simulink model "pitch_sim"  (R2025b)
settings: Solver=FixedStepAuto  StartTime=0.0  StopTime=15  FixedStep=0.0001  RelTol=1e-3
values from neighbouring files (symbols this model uses):
  A = [M1\M2; 0 0 1 0]    [Final_sim.m]    (also in hw2.m = 20; linear_fit_hw.m = [1 900 900^2; off_highway_tiremodel.m = [0.67 0.65 0.52 0.53 0.88]; sim3.m = [ 0 0 1 0)
  B = [M1\M3; 0 0]    [Final_sim.m]    (also in off_highway_tiremodel.m = 1.01*(100/Fz(1))*exp(0.14)-0.8401; sim3.m = [ 0     0; sim4.m = [(C1/m); (x1*C1)/(I)])
  C = [ 1 0 0 0 ... (first row only)    [sim3.m]    (also in sim4.m = eye(2,2))
  D = ddphiF+ddphiR    (= 1500)    [Final_sim.m]    (also in Final_sim_nonlinear.m; sim3.m = zeros(2,2); sim4.m = zeros(2,1))
settings Model: Creator=elija  LastModifiedBy=elija

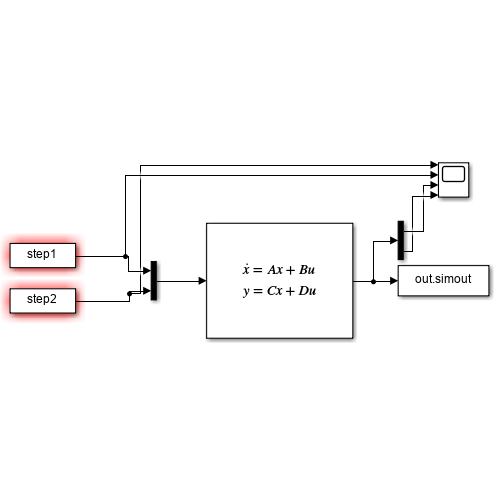
[thumbnail: Simulink's stored preview of the top-level diagram]
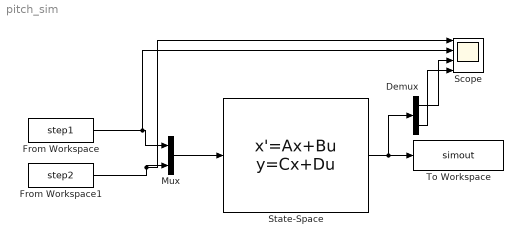
== system pitch_sim ==
  Demux : Demux  Outputs=2
  From Workspace : FromWorkspace  VariableName=step1  SampleTime=-1
  From Workspace1 : FromWorkspace  VariableName=step2  SampleTime=-1
  Mux : Mux  Inputs=2
  Scope : Scope  NumInputPorts=4
      settings: ActiveDisplayYMinimum=-1.0490987550558657  ActiveDisplayYMaximum=0.762340530638132
  State-Space : StateSpace  A=A  B=B  C=C  D=D  InitialCondition=0
  To Workspace : ToWorkspace  VariableName=simout  SaveFormat=Timeseries  SampleTime=-1
  wires:
  From Workspace/1 -> Scope/2, Mux/1
  State-Space/1 -> Demux/1, To Workspace/1
  From Workspace1/1 -> Scope/1, Mux/2
  Mux/1 -> State-Space/1
  Demux/1 -> Scope/3
  Demux/2 -> Scope/4
